simulink model "model_1"  (R2021b)
settings: Solver=VariableStepAuto  StartTime=0.0  StopTime=2.99  RelTol=1e-3
values from neighbouring files (symbols this model uses):
  A = [-6, 0, 0, 0; 0, 8,  0, 0; 0, 0, 2, 5; 0, 0, -5, 2]    [task_1.m]    (also in task_2.m = [0, 7, 0, 0; -7, 0,  0, 0; 0, 0, 0, 1; 0, 0, -1, 0]; task_3.m = [5, -9, -7, 1; -9, 5,  -1, 7; -7, -1, 5, 9; 1, 7, 9, 5])
  B = [0; 1; 9; 2]    [task_1.m]    (also in task_2.m = [0; 0; 0; 0]; task_3.m = [3; 3; 1; 3])
  C = [1, 0, 0, 0; 0, 1, 0, 0; 0, 0, 1, 0; 0, 0, 0, 1]    [task_1.m]    (also in task_2.m = [0, 5, 5, 0]; task_3.m = [2, -2, 2, 2; -2, 4, 2, 4])
  D = zeros(4, 1)    [task_1.m]    (also in task_2.m = 0; task_3.m = zeros(2, 1))
  K = - Y1 * inv(P)    [task_1.m]
  x_0 = [1; 1; 1; 1]    [task_1.m]    (also in task_2.m = [2; 0; 0; -1])
settings Model: Creator=vital  LastModifiedBy=vital

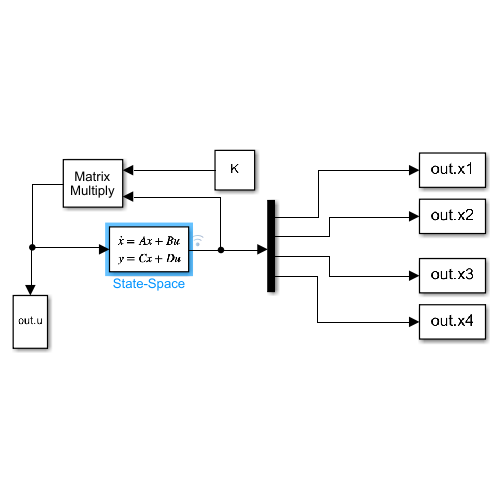
[thumbnail: Simulink's stored preview of the top-level diagram]
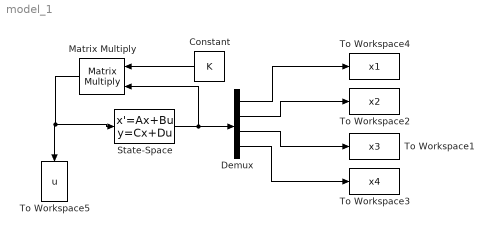
== system model_1 ==
  Constant : Constant  Value=K  VectorParams1D=off
  Demux : Demux
  Matrix Multiply : Product  Multiplication=Matrix(*)
  State-Space : StateSpace  A=A  B=B  C=C  D=D  InitialCondition=x_0  ParameterTunability=Unconstrained
  To Workspace1 : ToWorkspace  VariableName=x3  SaveFormat=Timeseries  SampleTime=-1
  To Workspace2 : ToWorkspace  VariableName=x2  SaveFormat=Timeseries  SampleTime=-1
  To Workspace3 : ToWorkspace  VariableName=x4  SaveFormat=Timeseries  SampleTime=-1
  To Workspace4 : ToWorkspace  VariableName=x1  SaveFormat=Timeseries  SampleTime=0.00001
  To Workspace5 : ToWorkspace  VariableName=u  SaveFormat=Timeseries  SampleTime=-1
  wires:
  State-Space/1 -> Matrix Multiply/2, Demux/1
  Demux/1 -> To Workspace4/1
  Demux/2 -> To Workspace2/1
  Demux/3 -> To Workspace1/1
  Demux/4 -> To Workspace3/1
  Constant/1 -> Matrix Multiply/1
  Matrix Multiply/1 -> State-Space/1, To Workspace5/1
